simulink model "PARTD_MSE452_Lab1_3L_VSI_samplemodel_r2022a"  (R2022a)
settings: Solver=ode23t  StartTime=0.0  StopTime=0.2  MaxStep=1e-5  RelTol=1e-3  EnableMultiTasking=on
InitFcn:
  | ma=0.3
  | f1=20
  | T1=1/f1
  | fs=900
  | Ts=1/fs
undefined symbols (not defined in the file): amp, f
libraries: spsDiodeLib x18, spsIdealSwitchLib x12, spsDCVoltageSourceLib x2, spsTriangleGeneratorLib x2, spsVoltageMeasurementLib x2, spsCurrentMeasurementLib x1, spsThreePhaseSeriesRLCBranchLib x1, spspowerguiLib x1
settings Model: Creator=Jason  LastModifiedBy=mitch
settings SolverCC: AlgebraicLoopSolver=TrustRegion
settings DataIOCC: LimitDataPoints=on  SaveFormat=Array  SignalLoggingSaveFormat=ModelDataLogs  ReturnWorkspaceOutputs=off
settings OptimizationCC: ExpressionDepthLimit=2147483647  InitFltsAndDblsToZero=on  LifeSpan=inf
settings DebuggingCC: SaveWithParameterizedLinksMsg=none  UnderspecifiedInitializationDetection=Classic  MergeDetectMultiDrivingBlocksExec=none  SignalResolutionControl=TryResolveAllWithWarning  SolverPrmCheckMsg=warning  MultiTaskDSMMsg=warning  MultiTaskCondExecSysMsg=none  FcnCallInpInsideContextMsg=warning  UnconnectedInputMsg=warning  UnconnectedOutputMsg=warning  UnconnectedLineMsg=warning  StateNameClashWarn=warning  SFUnexpectedBacktrackingDiag=warning  SFNoUnconditionalDefaultTransitionDiag=warning  SFExecutionAtInitializationDiag=none  ArithmeticOperatorsInVariantConditions=warning
settings HardwareCC: ProdBitPerPointer=32  ProdBitPerSizeT=32  ProdBitPerPtrDiffT=32  ProdLargestAtomicFloat=None  ProdIntDivRoundTo=Undefined  ProdEndianess=Unspecified  ProdWordSize=32  ProdHWDeviceType=32-bit Generic
settings ModelReferenceCC: PropagateSignalLabelsOutOfModel=off
settings SFSimCC: SimUseLocalCustomCode=off  CustomCodeUndefinedFunction=UseInterfaceOnly
settings RTWCC: RTWUseLocalCustomCode=off
settings CodeAppCC: StateflowObjectComments=on
settings GRTTargetCC: TargetFcnLib=ansi_tfl_tmw.mat  TargetLangStandard=C89/C90 (ANSI)  CombineOutputUpdateFcns=off  GRTInterface=on
settings ConfigComp: CovMetricSettings=dw  CovSaveCumulativeToWorkspaceVar=on  CovSaveSingleToWorkspaceVar=on  CovExternalEMLEnable=off
settings SimscapeCC: SimscapeNormalizeSystem=off

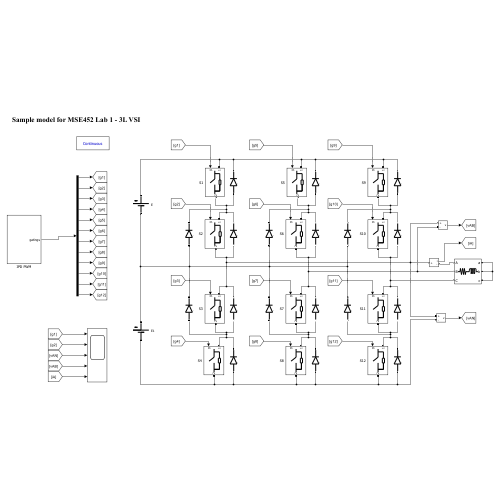
[thumbnail: Simulink's stored preview of the top-level diagram]
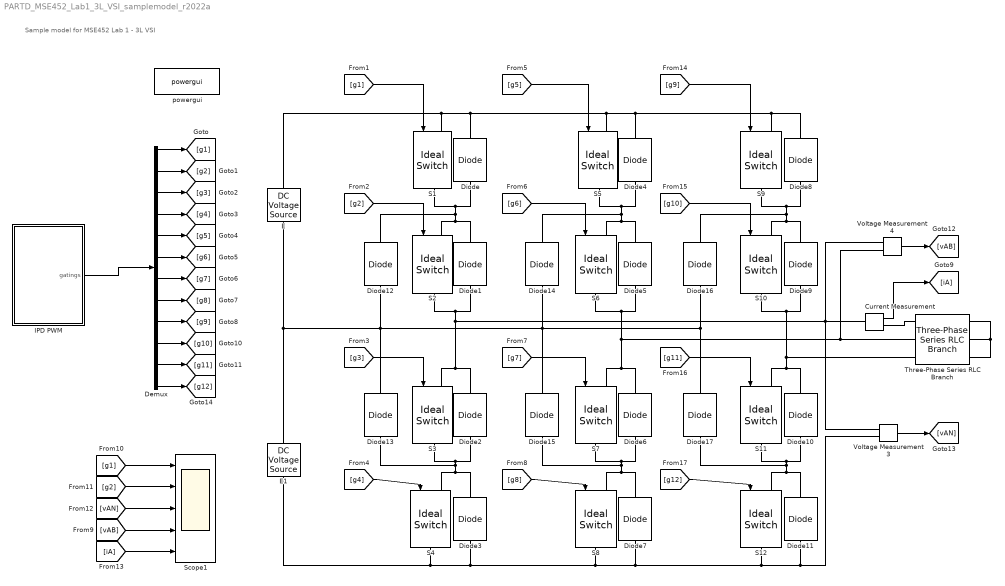
== system PARTD_MSE452_Lab1_3L_VSI_samplemodel_r2022a ==
  note: Sample model for MSE452 Lab 1 - 3L VSI
  Current Measurement : spsCurrentMeasurementLib/Current Measurement  PhasorSimulation=off  OutputType=Complex  PSBequivalent=0
  Demux : Demux  Outputs=12
  Diode{,1..17} (18 alike) : spsDiodeLib/Diode  Ron=0.001  Lon=0  Vf=0  IC=0  UseSnubber=off  Rs=inf  Cs=0  Measurements=off
  E : spsDCVoltageSourceLib/DC Voltage Source  Amplitude=5388.88  Measurements=None
  E1 : spsDCVoltageSourceLib/DC Voltage Source  Amplitude=5388.88  Measurements=None
  IPD PWM : Subsystem
  S{1..12} (12 alike) : spsIdealSwitchLib/Ideal Switch  Ron=0.001  Lon=0  IC=0  Rs=1e5  Cs=inf  Measurements=off
  Scope1 : Scope  NumInputPorts=5
  Three-Phase Series RLC Branch : spsThreePhaseSeriesRLCBranchLib/Three-Phase Series RLC Branch  LConnTagsString=A|B|C  RConnTagsString=A|B|C  BranchType=RL  Resistance=7.8408  Inductance=10.076e-3  Capacitance=1e-6  Measurements=None
  Voltage Measurement3 : spsVoltageMeasurementLib/Voltage Measurement  PhasorSimulation=off  OutputType=Complex  PSBequivalent=0
  Voltage Measurement4 : spsVoltageMeasurementLib/Voltage Measurement  PhasorSimulation=off  OutputType=Complex  PSBequivalent=0
  powergui : spspowerguiLib/powergui  SimulationMode=Continuous  SampleTime=0  frequency=60  Iterations=50  frequencyindice=0  Pbase=100e6  ErrMax=1e-4  UnitsV=kV  UnitsW=MW  buscounter=0  FunctionMessages=off  echomessages=off  EnableUseOfTLC=off  CurrentSourceSwitches=on  DisableSnubberDevices=off  DisableRonSwitches=off  DisableVfSwitches=off  DisplayEquations=off  AutomaticDiscreteSolvers=off  SolverType=Tustin  Interpol=off  ExternalGateDelay=off  methode=off  Ts=0  x0status=blocks  SPID=off  SwTol=0  HookPort=off  NonlinearTolerance=1e-4  nMaxIteration=100  ContinueOnMaxIteration=off  RestoreLinks=warning  ResistiveCurrentMeasurement=off  Frange=[0:2:500]  Ylog=off  Xlog=on  ShowGrid=off  save=off  variable=ZData  structure=npc  ZoomFFT=on  StartTime=1/20  cycles=2  DisplayStyle=3  fundamental=20  FreqAxis=on  MaxFrequency=20*300  frequencyindicesteady=1  RmsSteady=1  display=off
  wires:
  Demux/1 -> [g1]
  Demux/2 -> [g2]
  Demux/3 -> [g3]
  Demux/4 -> [g4]
  Demux/5 -> [g5]
  Demux/6 -> [g6]
  Demux/7 -> [g7]
  Demux/8 -> [g8]
  Demux/9 -> [g9]
  IPD PWM/1(gatings) -> Demux/1
  Voltage Measurement4/1 -> [vAB]
  Voltage Measurement3/1 -> [vAN]
  [vAB] -> Scope1/4
  [g1] -> Scope1/1
  [g2] -> Scope1/2
  [vAN] -> Scope1/3
  [iA] -> Scope1/5
  Current Measurement/1 -> [iA]
  Demux/10 -> [g10]
  Demux/11 -> [g11]
  Demux/12 -> [g12]
  [g1] -> S1/1
  [g2] -> S2/1
  [g3] -> S3/1
  [g4] -> S4/1
  [g5] -> S5/1
  [g6] -> S6/1
  [g7] -> S7/1
  [g8] -> S8/1
  [g9] -> S9/1
  [g10] -> S10/1
  [g11] -> S11/1
  [g12] -> S12/1
  connections:
  S5/LConn1 -- S1/LConn1 -- E/RConn1 -- Diode/RConn1 -- Diode4/RConn1 -- S9/LConn1 -- Diode8/RConn1
  Diode12/RConn1 -- S1/RConn1 -- Diode/LConn1 -- S2/LConn1 -- Diode1/RConn1
  Current Measurement/LConn1 -- Voltage Measurement4/LConn1 -- Voltage Measurement3/LConn1 -- S3/LConn1 -- Diode2/RConn1 -- Diode1/LConn1 -- S2/RConn1
  S3/RConn1 -- Diode2/LConn1 -- Diode3/RConn1 -- S4/LConn1 -- Diode13/LConn1
  Voltage Measurement3/LConn2 -- S12/RConn1 -- S4/RConn1 -- E1/LConn1 -- Diode3/LConn1 -- S8/RConn1 -- Diode7/LConn1 -- Diode11/LConn1
  Diode12/LConn1 -- E/LConn1 -- E1/RConn1 -- Diode13/RConn1 -- Diode14/LConn1 -- Diode15/RConn1 -- Diode16/LConn1 -- Diode17/RConn1
  S5/RConn1 -- Diode5/RConn1 -- S6/LConn1 -- Diode14/RConn1 -- Diode4/LConn1
  Three-Phase Series RLC Branch/LConn2 -- Diode6/RConn1 -- S7/LConn1 -- S6/RConn1 -- Diode5/LConn1 -- Voltage Measurement4/LConn2
  Diode6/LConn1 -- S7/RConn1 -- S8/LConn1 -- Diode7/RConn1 -- Diode15/LConn1
  S9/RConn1 -- Diode8/LConn1 -- S10/LConn1 -- Diode9/RConn1 -- Diode16/RConn1
  Three-Phase Series RLC Branch/LConn3 -- S11/LConn1 -- Diode10/RConn1 -- Diode9/LConn1 -- S10/RConn1
  S11/RConn1 -- Diode10/LConn1 -- Diode11/RConn1 -- S12/LConn1 -- Diode17/LConn1
  Three-Phase Series RLC Branch/RConn1 -- Three-Phase Series RLC Branch/RConn2 -- Three-Phase Series RLC Branch/RConn3
  Three-Phase Series RLC Branch/LConn1 -- Current Measurement/RConn1

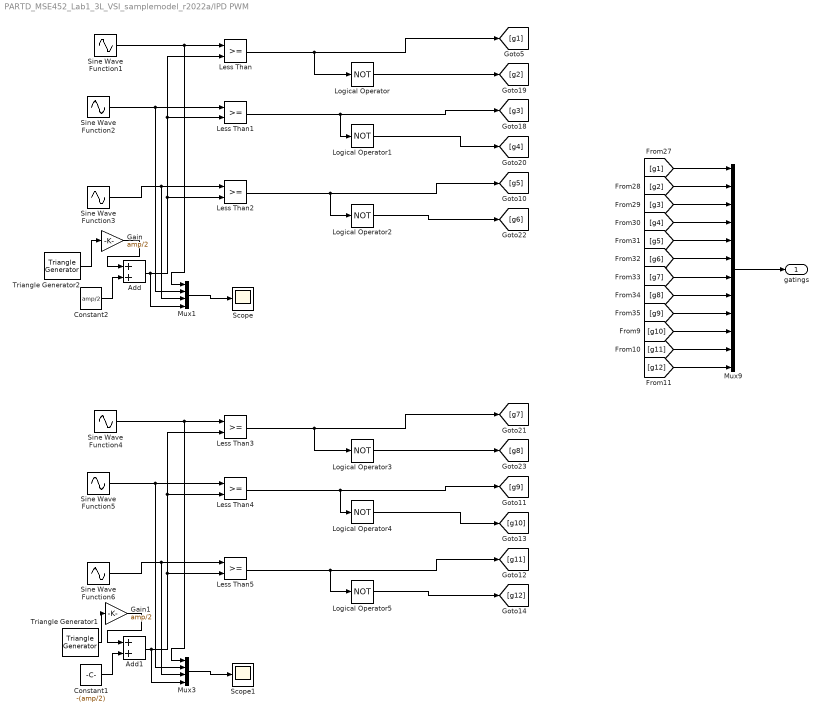
== system PARTD_MSE452_Lab1_3L_VSI_samplemodel_r2022a/IPD PWM ==
  Add : Sum
  Add1 : Sum
  Constant1 : Constant  Value=-(amp/2)
  Constant2 : Constant  Value=amp/2
  Gain : Gain  Gain=amp/2
  Gain1 : Gain  Gain=amp/2
  Less Than{,1..5} (6 alike) : RelationalOperator  OutDataTypeStr=boolean  RndMeth=Simplest  InputSameDT=off
  Logical Operator{,1..5} (6 alike) : Logic  Operator=NOT  AllPortsSameDT=off  OutDataTypeStr=boolean
  Mux1 : Mux
  Mux3 : Mux
  Mux9 : Mux  Inputs=12
  Scope : Scope
  Scope1 : Scope
  Sine Wave Function1 : Sin  Amplitude=0.4  Frequency=2*pi*f  SampleTime=0
  Sine Wave Function2 : Sin  Amplitude=0.4  Frequency=2*pi*f  Phase=-2*pi/3  SampleTime=0
  Sine Wave Function3 : Sin  Amplitude=0.4  Frequency=2*pi*f  Phase=2*pi/3  SampleTime=0
  Sine Wave Function4 : Sin  Amplitude=0.4  Frequency=2*pi*f  SampleTime=0
  Sine Wave Function5 : Sin  Amplitude=0.4  Frequency=2*pi*f  Phase=-2*pi/3  SampleTime=0
  Sine Wave Function6 : Sin  Amplitude=0.4  Frequency=2*pi*f  Phase=2*pi/3  SampleTime=0
  Triangle Generator1 : spsTriangleGeneratorLib/Triangle Generator  Freq=720  Phase=90  Ts=0
  Triangle Generator2 : spsTriangleGeneratorLib/Triangle Generator  Freq=720  Phase=90  Ts=0
  gatings : Outport  VectorParamsAs1DForOutWhenUnconnected=off
  wires:
  Mux9/1 -> gatings/1
  [g1] -> Mux9/1
  [g2] -> Mux9/2
  [g3] -> Mux9/3
  [g4] -> Mux9/4
  [g5] -> Mux9/5
  [g6] -> Mux9/6
  [g7] -> Mux9/7
  [g8] -> Mux9/8
  [g9] -> Mux9/9
  [g10] -> Mux9/10
  [g11] -> Mux9/11
  [g12] -> Mux9/12
  Mux1/1 -> Scope/1
  Logical Operator1/1 -> [g4]
  Sine Wave Function2/1 -> Mux1/2, Less Than1/1
  Logical Operator2/1 -> [g6]
  Sine Wave Function1/1 -> Mux1/1, Less Than/1
  Less Than/1 -> [g1], Logical Operator/1
  Less Than1/1 -> [g3], Logical Operator1/1
  Logical Operator/1 -> [g2]
  Less Than2/1 -> [g5], Logical Operator2/1
  Sine Wave Function3/1 -> Mux1/3, Less Than2/1
  Mux3/1 -> Scope1/1
  Logical Operator4/1 -> [g10]
  Sine Wave Function5/1 -> Mux3/2, Less Than4/1
  Logical Operator5/1 -> [g12]
  Sine Wave Function4/1 -> Mux3/1, Less Than3/1
  Less Than3/1 -> [g7], Logical Operator3/1
  Less Than4/1 -> [g9], Logical Operator4/1
  Logical Operator3/1 -> [g8]
  Less Than5/1 -> [g11], Logical Operator5/1
  Sine Wave Function6/1 -> Mux3/3, Less Than5/1
  Constant1/1 -> Add1/2
  Add1/1 -> Mux3/4, Less Than3/2, Less Than4/2, Less Than5/2
  Constant2/1 -> Add/2
  Add/1 -> Mux1/4, Less Than2/2, Less Than/2, Less Than1/2
  Triangle Generator2/1 -> Gain/1
  Gain/1 -> Add/1
  Triangle Generator1/1 -> Gain1/1
  Gain1/1 -> Add1/1
